simulink model "uz_ResonantController_2021a"  (R2021a)
settings: Solver=FixedStepDiscrete  StartTime=0.0  StopTime=0.01  RelTol=1e-3  EnableMultiTasking=on
PreLoadFcn:
  | uz_setCodegenPaths
model workspace (MATLAB code in the model file):
  | cmdLim = Simulink.Parameter;
  | cmdLim.Value = 15;
  | cmdLim.Description = 'Limit for controlling the maximum surface command angle.';
  | cmdLim.Min = 0;
  | cmdLim.Max = 90;
  | cmdLim.DocUnits = 'deg';
  | 
  | dispGain = Simulink.Parameter;
  | dispGain.Value = 0.75;
  | dispGain.Description = 'Gain applied to the displacement error.';
  | dispGain.Min = 0;
  | dispGain.Max = [];
  | dispGain.DocUnits = 'deg/sec/deg';
  | 
  | dispLim = Simulink.Parameter;
  | dispLim.Value = 30;
  | dispLim.Description = 'Limit for controlling the maximum commanded angle.';
  | dispLim.Min = 0;
  | dispLim.Max = 180;
  | dispLim.DocUnits = 'deg';
  | 
  | intGain = Simulink.Parameter;
  | intGain.Value = 0.5;
  | intGain.Description = 'Gain applied to the integral error.';
  | intGain.Min = 0;
  | intGain.Max = [];
  | intGain.DocUnits = 'deg/sec/deg/sec';
  | 
  | intLim = Simulink.Parameter;
  | intLim.Value = 5;
  | intLim.Description = 'Limit for controlling the maximum commanded angle.';
  | intLim.Min = 0;
  | intLim.Max = 90;
  | intLim.DocUnits = 'deg';
  | 
  | rateGain = Simulink.Parameter;
  | rateGain.Value = 2;
  | rateGain.Description = 'Gain applied to the rate error.';
  | rateGain.Min = 0;
  | rateGain.Max = [];
  | rateGain.DocUnits = 'deg/deg/sec';
  | 
  | rateLim = Simulink.Parameter;
  | rateLim.Value = 6;
  | rateLim.Description = 'Limit for controlling the maximum commanded angle.';
  | rateLim.Min = 0;
  | rateLim.Max = 180;
  | rateLim.DocUnits = 'deg/sec';
  | 
  | hdgGain = Simulink.Parameter;
  | hdgGain.Value = 0.015;
settings Model: RequirementInfo={} %GIDa_fe9045fd_0412_4b6e_8206_617cc20e6fde  FPTRunName=Active  Creator=ts  LastModifiedBy=micha
settings SolverCC: AlgebraicLoopSolver=TrustRegion  PositivePriorityOrder=on  AutoInsertRateTranBlk=on
settings DataIOCC: SaveOutput=off  SignalLogging=off  DSMLogging=off  SaveTime=off
settings OptimizationCC: DefaultParameterBehavior=Inlined  UseDivisionForNetSlopeComputation=on  GainParamInheritBuiltInType=on  UseFloatMulNetSlope=on  UseSpecifiedMinMax=on  InlineInvariantSignals=on  PassReuseOutputArgsAs=Individual arguments  NoFixptDivByZeroProtection=on  EfficientFloat2IntCast=on  LifeSpan=1  MaxStackSize=64  OptimizeBlockOrder=speed  DifferentSizesBufferReuse=on  EfficientTunableParamExpr=on
settings DebuggingCC: AllowSymbolicDim=off  SFUnexpectedBacktrackingDiag=warning  SFNoUnconditionalDefaultTransitionDiag=warning  SFExecutionAtInitializationDiag=none  ArithmeticOperatorsInVariantConditions=warning
settings HardwareCC: ProdBitPerPointer=32  ProdBitPerSizeT=32  ProdBitPerPtrDiffT=32  ProdLargestAtomicInteger=Long  ProdLargestAtomicFloat=Double  ProdWordSize=32  ProdLongLongMode=on  ProdHWDeviceType=ARM Compatible->ARM Cortex-R  HardwareBoardFeatureSet=SoCBlockset
settings SFSimCC: MATLABDynamicMemAlloc=off
settings RTWCC: SystemTargetFile=ert.tlc  GenCodeOnly=on  TemplateMakefile=ert_default_tmf  GenerateReport=on  BuildConfiguration=Faster Runs  IncludeHyperlinkInReport=on  GenerateCodeMetricsReport=on  CheckMdlBeforeBuild=Warning
settings CodeAppCC: ForceParamTrailComments=on  IgnoreCustomStorageClasses=off  OperatorAnnotations=on  SimulinkDataObjDesc=on  SFDataObjDesc=on  MATLABFcnDesc=on  InsertBlockDesc=on  StateflowObjectComments=on  MATLABSourceComments=on  EnableCustomComments=on  ReqsInCode=on
settings ERTTargetCC: TargetLangStandard=C99 (ISO)  CodeReplacementLibrary=GNU C99 extensions  MultiwordLength=2048  IncludeMdlTerminateFcn=off  CombineSignalStateStructs=on  SuppressErrorStatus=on  IncludeFileDelimiter=UseQuote  SupportAbsoluteTime=off  CodeInterfacePackaging=Reusable function  SupportNonFinite=off  RemoveResetFunc=off  InlinedParameterPlacement=NonHierarchical  MultiInstanceErrorCode=Warning  RootIOFormat=Part of model data structure  ERTCustomFileTemplate=example_file_process.tlc  GlobalDataDefinition=InSourceFile  GlobalDataReference=InSourceFile  ERTFilePackagingFormat=CompactWithDataFile
settings ConfigComp: CovScope=ReferencedModels  CovSaveName=covdata_rollAP  CovMetricSettings=dcmtrwe  CovHTMLOptions=-sRT=1 -aTS=1 -bRG=1 -bTC=1 -hTR=1 -nFC=0 -scm=1 -bcm=1 -xEv=0  CovSaveCumulativeToWorkspaceVar=on  CovSaveSingleToWorkspaceVar=on  CovCumulativeVarName=covCumulativeData_rollAP  CovReportOnPause=off  CovExternalEMLEnable=off  CovSFcnEnable=off

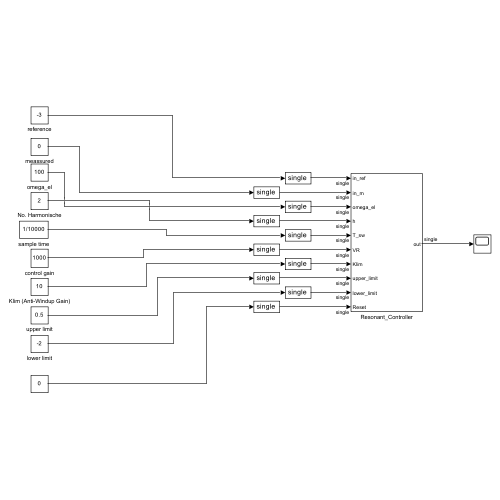
[thumbnail: Simulink's stored preview of the top-level diagram]
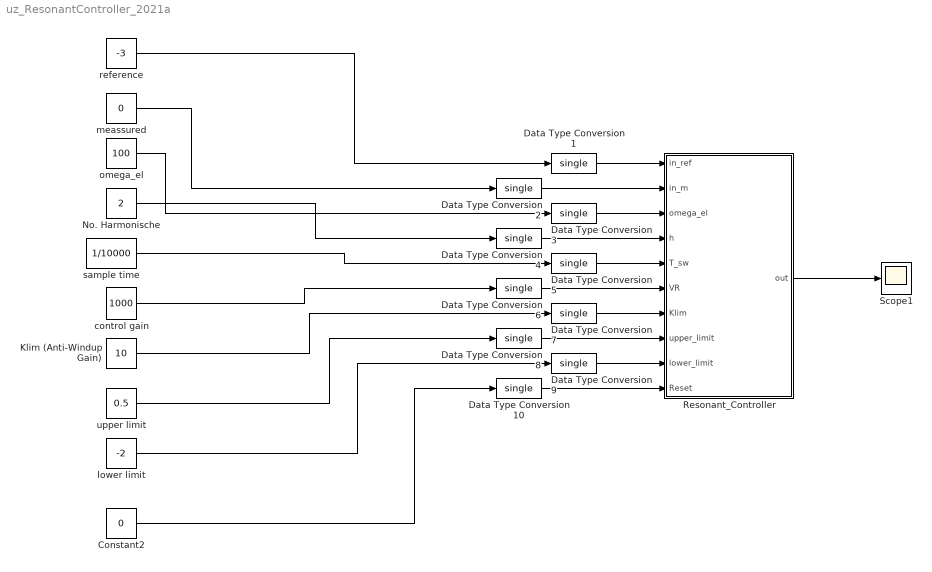
== system uz_ResonantController_2021a ==
  Constant2 : Constant  Value=0
  Data Type Conversion{1..10} (10 alike) : DataTypeConversion  OutDataTypeStr=single
  Klim (Anti-Windup Gain) : Constant  Value=10
  No. Harmonische : Constant  Value=2
  Resonant_Controller : Subsystem
  Scope1 : Scope
  control gain : Constant  Value=1000
  lower limit : Constant  Value=-2
  meassured : Constant  Value=0
  omega_el : Constant  Value=100
  reference : Constant  Value=-3
  sample time : Constant  Value=1/10000
  upper limit : Constant  Value=0.5
  wires:
  sample time/1 -> Data Type Conversion5/1
  No. Harmonische/1 -> Data Type Conversion4/1
  reference/1 -> Data Type Conversion1/1
  meassured/1 -> Data Type Conversion2/1
  control gain/1 -> Data Type Conversion6/1
  omega_el/1 -> Data Type Conversion3/1
  Resonant_Controller/1(out) -> Scope1/1
  Klim (Anti-Windup Gain)/1 -> Data Type Conversion7/1
  upper limit/1 -> Data Type Conversion8/1
  lower limit/1 -> Data Type Conversion9/1
  Constant2/1 -> Data Type Conversion10/1
  Data Type Conversion1/1 -> Resonant_Controller/1(in_ref)
  Data Type Conversion2/1 -> Resonant_Controller/2(in_m)
  Data Type Conversion3/1 -> Resonant_Controller/3(omega_el)
  Data Type Conversion4/1 -> Resonant_Controller/4(h)
  Data Type Conversion5/1 -> Resonant_Controller/5(T_sw)
  Data Type Conversion6/1 -> Resonant_Controller/6(VR)
  Data Type Conversion7/1 -> Resonant_Controller/7(Klim)
  Data Type Conversion8/1 -> Resonant_Controller/8(upper_limit)
  Data Type Conversion9/1 -> Resonant_Controller/9(lower_limit)
  Data Type Conversion10/1 -> Resonant_Controller/10(Reset)

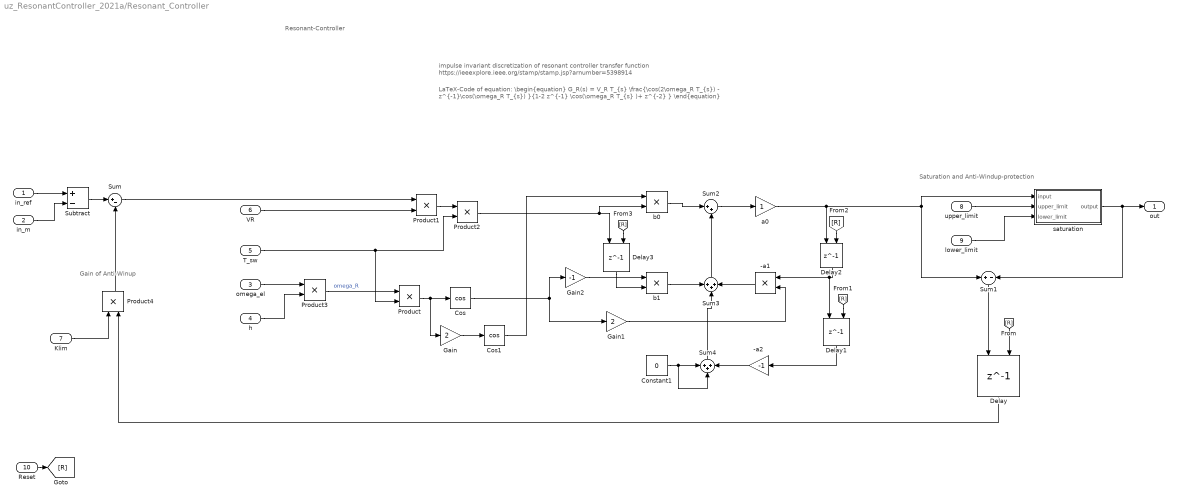
== system uz_ResonantController_2021a/Resonant_Controller ==
  note: Gain of Anti-Winup
  note: Saturation and Anti-Windup-protection
  note: Resonant-Controller
  note: impulse invariant discretization of resonant controller transfer function
      | https://ieeexplore.ieee.org/stamp/stamp.jsp?arnumber=5398914
  note: LaTeX-Code of equation:
      | \begin{equation}
      | 	G_R(s) = V_R T_{s} \frac{\cos(2\omega_R T_{s}) - z^{-1}\cos(\omega_R T_{s}) }{1-2 z^{-1} \cos(\omega_R T_{s} )+ z^{-2} }
      | \end{equation}
  in_ref : Inport  OutDataTypeStr=single
  in_m : Inport  Port=2  OutDataTypeStr=single
  omega_el : Inport  Port=3  OutDataTypeStr=single
  h : Inport  Port=4  OutDataTypeStr=single
  T_sw : Inport  Port=5  OutDataTypeStr=single
  VR : Inport  Port=6  OutDataTypeStr=single
  Klim : Inport  Port=7  OutDataTypeStr=single
  upper_limit : Inport  Port=8  OutDataTypeStr=single
  lower_limit : Inport  Port=9  OutDataTypeStr=single
  Reset : Inport  Port=10  OutDataTypeStr=single
  -a1 : Product
  -a2 : Gain  Gain=-1
  Constant1 : Constant  Value=0  OutDataTypeStr=single
  Cos : Trigonometry  Operator=cos
  Cos1 : Trigonometry  Operator=cos
  Delay{,1..3} (4 alike) : Delay  DelayLength=1  InitialCondition=0  ExternalReset=Level hold  SampleTime=1/10000
      settings: InputPortMap=u0,r5
  Gain : Gain  Gain=2
  Gain1 : Gain  Gain=2
  Gain2 : Gain  Gain=-1
  Product{,1..3} (4 alike) : Product
  Product4 : Product  OutDataTypeStr=single
  Subtract : Sum  Inputs=+-
  Sum : Sum  Inputs=|+-
  Sum1 : Sum  Inputs=+|-
  Sum2 : Sum  Inputs=|++
  Sum3 : Sum  Inputs=+++
  Sum4 : Sum  Inputs=+++
  a0 : Gain  OutDataTypeStr=single
  b0 : Product  OutDataTypeStr=single
  b1 : Product
  saturation : MATLAB Function  TreatAsAtomicUnit=on
  out : Outport  OutDataTypeStr=single
  wires:
  Cos/1 -> Gain1/1, Gain2/1
  T_sw/1 -> Product/2, Product2/2
  Product/1 -> Gain/1, Cos/1
  Gain/1 -> Cos1/1
  Sum4/1 -> Sum3/2
  b1/1 -> Sum3/1
  -a1/1 -> Sum3/3
  Delay2/1 -> -a1/1, Delay1/1
  Delay1/1 -> -a2/1
  -a2/1 -> Sum4/3
  Delay3/1 -> b1/2
  b0/1 -> Sum2/1
  Sum3/1 -> Sum2/2
  Sum2/1 -> a0/1
  a0/1 -> saturation/1(input), Sum1/1, Delay2/1
  Constant1/1 -> Sum4/1, Sum4/2
  Gain1/1 -> -a1/2
  Product1/1 -> Product2/1
  Product2/1 -> Delay3/1, b0/2
  omega_el/1 -> Product3/1
  Product3/1 -> Product/1  "omega_R"
  h/1 -> Product3/2
  Cos1/1 -> b0/1
  Gain2/1 -> b1/1
  VR/1 -> Product1/2
  in_ref/1 -> Subtract/1
  in_m/1 -> Subtract/2
  Subtract/1 -> Sum/1
  Sum/1 -> Product1/1
  Product4/1 -> Sum/2
  Klim/1 -> Product4/1
  Sum1/1 -> Delay/1
  saturation/1(output) -> Sum1/2, out/1
  upper_limit/1 -> saturation/2(upper_limit)
  lower_limit/1 -> saturation/3(lower_limit)
  Delay/1 -> Product4/2
  Reset/1 -> [R]
  [R] -> Delay/2
  [R] -> Delay1/2
  [R] -> Delay2/2
  [R] -> Delay3/2

== matlab function uz_ResonantController_2021a/Resonant_Controller/saturation ==
  data: input input; output output; upper_limit input; lower_limit input
function output = fcn(input, upper_limit, lower_limit)

output = input;

if (input > upper_limit)
    output = upper_limit;
end

if (input < lower_limit)
    output = lower_limit;
end
